simulink model "iff_sim"  (R2019b)
settings: Solver=VariableStepAuto  StartTime=0.0  StopTime=T  FixedStep=0.001  MaxStep=0.001  RelTol=1e-3
values from neighbouring files (symbols this model uses):
  bsc = 17    [model.mat]    (also in model_data.m)
  d_r = [0.01 0.01 0.01 0.01 0.01 0.01]    [model.mat]    (also in model_data.m = 0.01*ones(6,1))
  Fi_b_z = [0 2.09439510239 4.18879020479 1.0471975512 3.14159265359 5.23598775598]    [model.mat]    (also in model_data.m = [0;2/3;4/3;1/3;3/3;5/3]*pi)
  Fp = 148    [model.mat]    (also in model_data.m)
  ka = 11860000    [model.mat]    (also in model_data.m)
  Kd = 0    [ctc_data.m]
  Ki = 0    [ctc_data.m]
  Kp = 300    [ctc_data.m]
  ksc = 179000    [model.mat]    (also in model_data.m)
  l_r = [0.36 0.36 0.36 0.36 0.36 0.36]    [model.mat]    (also in model_data.m = 0.36*ones(6,1))
  la00 = 0.061    [model.mat]    (also in model_data.m)
  O_lb = [0 0 0 0 0 0]    [model.mat]    (also in model_data.m = [0;0;0;0;0;0])
  q_d = out_ik.q'    [ik_run.m]
  qt_d = out_ik.qt'    [ik_run.m]
  qtt_d = out_ik.qtt'    [ik_run.m]
  RMSforce = 35    [model.mat]
  s = out_ctc.s    [ctc_run.m]
  s_0 = s_d(:,:,1)    [ctc_run.m]    (also in iff_run.m)
  T = 1.5    [ctc_data.m]
  t_d = out_ik.t'    [ik_run.m]
  t_dist = 0.1    [model.mat]
  ts_noise = 1.6e-05    [model.mat]    (also in model_data.m)
  v_0 = v_d(:,:,1)    [ctc_run.m]    (also in iff_run.m)
  w_lb = 0.195    [model.mat]    (also in model_data.m)
  W_lb = 0.205    [model.mat]    (also in model_data.m)
  w_ub = 0.195    [model.mat]    (also in model_data.m)
  W_ub = 0.205    [model.mat]    (also in model_data.m)
undefined symbols (not defined in the file or in its folder): X, Y, Z
libraries: nesl_utility x282, sm_lib x208, dspindex x30, simulink x12, powerlib_meascontrol x1
(part 14 of 14)

== system iff_sim/High-authority control/CTC/computed torque control/bases + rods/upper base/O_ub -> H_4 ==
  rot z : sm_lib/Frames and Transforms/Rigid Transform  TranslationMethod=None  TranslationStandardOffset=0  TranslationLengthUnit=m  TranslationStandardAxis=+Z  TranslationCartesianOffset=[0 0 0]  TranslationROffset=0  TranslationROffsetUnits=m  TranslationZOffset=0  TranslationZOffsetUnits=m  TranslationThetaOffset=0  TranslationThetaOffsetUnits=deg  RotationMethod=StandardAxis  RotationAngleUnits=rad  RotationStandardAxis=+Z  RotationAngle=Fi_b_z(4)  RotationArbitraryAxis=[0 0 1]  FollAlignAxisA=+X  BaseAlignAxisA=+Y  FollAlignAxisB=+Y  BaseAlignAxisB=+Z  RotationSequenceAxes=FollowerAxes  RotationSequence=XYX  RotationSequenceAngles=[0 0 0]  RotationSequenceAnglesUnits=deg  RotationMatrix=[1 0 0; 0 1 0; 0 0 1]
  trans z : sm_lib/Frames and Transforms/Rigid Transform  TranslationMethod=StandardAxis  TranslationStandardOffset=h_ub  TranslationLengthUnit=m  TranslationStandardAxis=-Z  TranslationCartesianOffset=[0 0 0]  TranslationROffset=0  TranslationROffsetUnits=m  TranslationZOffset=0  TranslationZOffsetUnits=m  TranslationThetaOffset=0  TranslationThetaOffsetUnits=deg  RotationMethod=None  RotationAngleUnits=deg  RotationStandardAxis=+Z  RotationAngle=0.0  RotationArbitraryAxis=[0 0 1]  FollAlignAxisA=+X  BaseAlignAxisA=+Y  FollAlignAxisB=+Y  BaseAlignAxisB=+Z  RotationSequenceAxes=FollowerAxes  RotationSequence=XYX  RotationSequenceAngles=[0 0 0]  RotationSequenceAnglesUnits=deg  RotationMatrix=[1 0 0; 0 1 0; 0 0 1]
  transl y : sm_lib/Frames and Transforms/Rigid Transform  TranslationMethod=StandardAxis  TranslationStandardOffset=w_ub/2  TranslationLengthUnit=m  TranslationStandardAxis=+Y  TranslationCartesianOffset=[0 0 0]  TranslationROffset=0  TranslationROffsetUnits=m  TranslationZOffset=0  TranslationZOffsetUnits=m  TranslationThetaOffset=0  TranslationThetaOffsetUnits=deg  RotationMethod=None  RotationAngleUnits=deg  RotationStandardAxis=+Z  RotationAngle=0.0  RotationArbitraryAxis=[0 0 1]  FollAlignAxisA=+X  BaseAlignAxisA=+Y  FollAlignAxisB=+Y  BaseAlignAxisB=+Z  RotationSequenceAxes=FollowerAxes  RotationSequence=XYX  RotationSequenceAngles=[0 0 0]  RotationSequenceAnglesUnits=deg  RotationMatrix=[1 0 0; 0 1 0; 0 0 1]
  O_ub : PMIOPort  Side=Left
  H_4 : PMIOPort  Port=2  Side=Right
  connections:
  trans z/LConn1 -- O_ub/RConn1
  trans z/RConn1 -- rot z/LConn1
  transl y/LConn1 -- rot z/RConn1
  transl y/RConn1 -- H_4/RConn1

== system iff_sim/High-authority control/CTC/computed torque control/bases + rods/upper base/O_ub -> H_5 ==
  rot z : sm_lib/Frames and Transforms/Rigid Transform  TranslationMethod=None  TranslationStandardOffset=0  TranslationLengthUnit=m  TranslationStandardAxis=+Z  TranslationCartesianOffset=[0 0 0]  TranslationROffset=0  TranslationROffsetUnits=m  TranslationZOffset=0  TranslationZOffsetUnits=m  TranslationThetaOffset=0  TranslationThetaOffsetUnits=deg  RotationMethod=StandardAxis  RotationAngleUnits=rad  RotationStandardAxis=+Z  RotationAngle=Fi_b_z(5)  RotationArbitraryAxis=[0 0 1]  FollAlignAxisA=+X  BaseAlignAxisA=+Y  FollAlignAxisB=+Y  BaseAlignAxisB=+Z  RotationSequenceAxes=FollowerAxes  RotationSequence=XYX  RotationSequenceAngles=[0 0 0]  RotationSequenceAnglesUnits=deg  RotationMatrix=[1 0 0; 0 1 0; 0 0 1]
  trans z : sm_lib/Frames and Transforms/Rigid Transform  TranslationMethod=StandardAxis  TranslationStandardOffset=h_ub  TranslationLengthUnit=m  TranslationStandardAxis=-Z  TranslationCartesianOffset=[0 0 0]  TranslationROffset=0  TranslationROffsetUnits=m  TranslationZOffset=0  TranslationZOffsetUnits=m  TranslationThetaOffset=0  TranslationThetaOffsetUnits=deg  RotationMethod=None  RotationAngleUnits=deg  RotationStandardAxis=+Z  RotationAngle=0.0  RotationArbitraryAxis=[0 0 1]  FollAlignAxisA=+X  BaseAlignAxisA=+Y  FollAlignAxisB=+Y  BaseAlignAxisB=+Z  RotationSequenceAxes=FollowerAxes  RotationSequence=XYX  RotationSequenceAngles=[0 0 0]  RotationSequenceAnglesUnits=deg  RotationMatrix=[1 0 0; 0 1 0; 0 0 1]
  transl y : sm_lib/Frames and Transforms/Rigid Transform  TranslationMethod=StandardAxis  TranslationStandardOffset=w_ub/2  TranslationLengthUnit=m  TranslationStandardAxis=+Y  TranslationCartesianOffset=[0 0 0]  TranslationROffset=0  TranslationROffsetUnits=m  TranslationZOffset=0  TranslationZOffsetUnits=m  TranslationThetaOffset=0  TranslationThetaOffsetUnits=deg  RotationMethod=None  RotationAngleUnits=deg  RotationStandardAxis=+Z  RotationAngle=0.0  RotationArbitraryAxis=[0 0 1]  FollAlignAxisA=+X  BaseAlignAxisA=+Y  FollAlignAxisB=+Y  BaseAlignAxisB=+Z  RotationSequenceAxes=FollowerAxes  RotationSequence=XYX  RotationSequenceAngles=[0 0 0]  RotationSequenceAnglesUnits=deg  RotationMatrix=[1 0 0; 0 1 0; 0 0 1]
  O_ub : PMIOPort  Side=Left
  H_5 : PMIOPort  Port=2  Side=Right
  connections:
  trans z/LConn1 -- O_ub/RConn1
  trans z/RConn1 -- rot z/LConn1
  transl y/LConn1 -- rot z/RConn1
  transl y/RConn1 -- H_5/RConn1

== system iff_sim/High-authority control/CTC/computed torque control/bases + rods/upper base/O_ub -> H_6 ==
  rot z : sm_lib/Frames and Transforms/Rigid Transform  TranslationMethod=None  TranslationStandardOffset=0  TranslationLengthUnit=m  TranslationStandardAxis=+Z  TranslationCartesianOffset=[0 0 0]  TranslationROffset=0  TranslationROffsetUnits=m  TranslationZOffset=0  TranslationZOffsetUnits=m  TranslationThetaOffset=0  TranslationThetaOffsetUnits=deg  RotationMethod=StandardAxis  RotationAngleUnits=rad  RotationStandardAxis=+Z  RotationAngle=Fi_b_z(6)  RotationArbitraryAxis=[0 0 1]  FollAlignAxisA=+X  BaseAlignAxisA=+Y  FollAlignAxisB=+Y  BaseAlignAxisB=+Z  RotationSequenceAxes=FollowerAxes  RotationSequence=XYX  RotationSequenceAngles=[0 0 0]  RotationSequenceAnglesUnits=deg  RotationMatrix=[1 0 0; 0 1 0; 0 0 1]
  trans z : sm_lib/Frames and Transforms/Rigid Transform  TranslationMethod=StandardAxis  TranslationStandardOffset=h_ub  TranslationLengthUnit=m  TranslationStandardAxis=-Z  TranslationCartesianOffset=[0 0 0]  TranslationROffset=0  TranslationROffsetUnits=m  TranslationZOffset=0  TranslationZOffsetUnits=m  TranslationThetaOffset=0  TranslationThetaOffsetUnits=deg  RotationMethod=None  RotationAngleUnits=deg  RotationStandardAxis=+Z  RotationAngle=0.0  RotationArbitraryAxis=[0 0 1]  FollAlignAxisA=+X  BaseAlignAxisA=+Y  FollAlignAxisB=+Y  BaseAlignAxisB=+Z  RotationSequenceAxes=FollowerAxes  RotationSequence=XYX  RotationSequenceAngles=[0 0 0]  RotationSequenceAnglesUnits=deg  RotationMatrix=[1 0 0; 0 1 0; 0 0 1]
  transl y : sm_lib/Frames and Transforms/Rigid Transform  TranslationMethod=StandardAxis  TranslationStandardOffset=w_ub/2  TranslationLengthUnit=m  TranslationStandardAxis=+Y  TranslationCartesianOffset=[0 0 0]  TranslationROffset=0  TranslationROffsetUnits=m  TranslationZOffset=0  TranslationZOffsetUnits=m  TranslationThetaOffset=0  TranslationThetaOffsetUnits=deg  RotationMethod=None  RotationAngleUnits=deg  RotationStandardAxis=+Z  RotationAngle=0.0  RotationArbitraryAxis=[0 0 1]  FollAlignAxisA=+X  BaseAlignAxisA=+Y  FollAlignAxisB=+Y  BaseAlignAxisB=+Z  RotationSequenceAxes=FollowerAxes  RotationSequence=XYX  RotationSequenceAngles=[0 0 0]  RotationSequenceAnglesUnits=deg  RotationMatrix=[1 0 0; 0 1 0; 0 0 1]
  O_ub : PMIOPort  Side=Left
  H_6 : PMIOPort  Port=2  Side=Right
  connections:
  trans z/LConn1 -- O_ub/RConn1
  trans z/RConn1 -- rot z/LConn1
  transl y/LConn1 -- rot z/RConn1
  transl y/RConn1 -- H_6/RConn1

== matlab function iff_sim/High-authority control/CTC/computed torque control/bases + rods/v_r,v_ub -> v ==
  data: v_1 input; v output; v_2 input; v_3 input; v_4 input; v_5 input; v_6 input; v_ub input
function v = fcn(v_1,v_2,v_3,v_4,v_5,v_6,v_ub)
    v = [v_1,v_2,v_3,v_4,v_5,v_6,v_ub];
end

== matlab function iff_sim/dynamic model/v -> qt ==
  data: v input; qt output
function qt = fcn(v)
    qt = zeros(18,1);
    for r = 1:1:6
        qt(((r-1)*2+1):((r-1)*2+2),1) = v(4:5,r);
    end
    qt(13:end) = v(:,7);
end

== matlab function iff_sim/High-authority control/CTC/computed torque control/desired cable vectors// lengths/cable 2/cable force and length ==
  data: pz input; F_c output; fz input; l_c output
function [F_c,l_c] = fcn(pz,fz)
    if pz < 0 
        F_c = fz;
    else
        F_c = -fz;
    end
    l_c = abs(pz);
end

== matlab function iff_sim/dynamic model/rods + bases/s_r,s_ub -> s ==
  data: s_1 input; s output; s_2 input; s_3 input; s_4 input; s_5 input; s_6 input; s_ub input
function s = fcn(s_1,s_2,s_3,s_4,s_5,s_6,s_ub)
    s = [s_1,s_2,s_3,s_4,s_5,s_6,s_ub];
end

== matlab function iff_sim/dynamic model/rods + bases/v_r,v_ub -> v ==
  data: v_1 input; v output; v_2 input; v_3 input; v_4 input; v_5 input; v_6 input; v_ub input
function v = fcn(v_1,v_2,v_3,v_4,v_5,v_6,v_ub)
    v = [v_1,v_2,v_3,v_4,v_5,v_6,v_ub];
end

== matlab function iff_sim/High-authority control/CTC/computed torque control/desired cable vectors// lengths/cable 1/cable force and length ==
  data: pz input; F_c output; fz input; l_c output
function [F_c,l_c] = fcn(pz,fz)
    if pz < 0 
        F_c = fz;
    else
        F_c = -fz;
    end
    l_c = abs(pz);
end

== matlab function iff_sim/High-authority control/CTC/computed torque control/desired cable vectors// lengths/cable 3/cable force and length ==
  data: pz input; F_c output; fz input; l_c output
function [F_c,l_c] = fcn(pz,fz)
    if pz < 0 
        F_c = fz;
    else
        F_c = -fz;
    end
    l_c = abs(pz);
end

== matlab function iff_sim/High-authority control/CTC/computed torque control/desired cable vectors// lengths/cable 4/cable force and length ==
  data: pz input; F_c output; fz input; l_c output
function [F_c,l_c] = fcn(pz,fz)
    if pz < 0 
        F_c = fz;
    else
        F_c = -fz;
    end
    l_c = abs(pz);
end

== matlab function iff_sim/High-authority control/CTC/computed torque control/desired cable vectors// lengths/cable 5/cable force and length ==
  data: pz input; F_c output; fz input; l_c output
function [F_c,l_c] = fcn(pz,fz)
    if pz < 0 
        F_c = fz;
    else
        F_c = -fz;
    end
    l_c = abs(pz);
end

== matlab function iff_sim/High-authority control/CTC/computed torque control/desired cable vectors// lengths/cable 6/cable force and length ==
  data: pz input; F_c output; fz input; l_c output
function [F_c,l_c] = fcn(pz,fz)
    if pz < 0 
        F_c = fz;
    else
        F_c = -fz;
    end
    l_c = abs(pz);
end

== matlab function iff_sim/High-authority control/CTC/computed torque control/desired cable vectors// lengths/cable 7/cable force and length ==
  data: pz input; F_c output; fz input; l_c output
function [F_c,l_c] = fcn(pz,fz)
    if pz < 0 
        F_c = fz;
    else
        F_c = -fz;
    end
    l_c = abs(pz);
end

== matlab function iff_sim/High-authority control/CTC/computed torque control/desired cable vectors// lengths/cable 8/cable force and length ==
  data: pz input; F_c output; fz input; l_c output
function [F_c,l_c] = fcn(pz,fz)
    if pz < 0 
        F_c = fz;
    else
        F_c = -fz;
    end
    l_c = abs(pz);
end

== matlab function iff_sim/High-authority control/CTC/computed torque control/desired cable vectors// lengths/cable 9/cable force and length ==
  data: pz input; F_c output; fz input; l_c output
function [F_c,l_c] = fcn(pz,fz)
    if pz < 0 
        F_c = fz;
    else
        F_c = -fz;
    end
    l_c = abs(pz);
end

== matlab function iff_sim/High-authority control/CTC/computed torque control/desired cable vectors// lengths/cable 10/cable force and length ==
  data: pz input; F_c output; fz input; l_c output
function [F_c,l_c] = fcn(pz,fz)
    if pz < 0 
        F_c = fz;
    else
        F_c = -fz;
    end
    l_c = abs(pz);
end

== matlab function iff_sim/High-authority control/CTC/computed torque control/desired cable vectors// lengths/cable 11/cable force and length ==
  data: pz input; F_c output; fz input; l_c output
function [F_c,l_c] = fcn(pz,fz)
    if pz < 0 
        F_c = fz;
    else
        F_c = -fz;
    end
    l_c = abs(pz);
end

== matlab function iff_sim/High-authority control/CTC/computed torque control/desired cable vectors// lengths/cable 12/cable force and length ==
  data: pz input; F_c output; fz input; l_c output
function [F_c,l_c] = fcn(pz,fz)
    if pz < 0 
        F_c = fz;
    else
        F_c = -fz;
    end
    l_c = abs(pz);
end

== matlab function iff_sim/High-authority control/CTC/computed torque control/desired cable vectors// lengths/cable 13/cable force and length ==
  data: pz input; F_c output; fz input; l_c output
function [F_c,l_c] = fcn(pz,fz)
    if pz < 0 
        F_c = fz;
    else
        F_c = -fz;
    end
    l_c = abs(pz);
end

== matlab function iff_sim/High-authority control/CTC/computed torque control/desired cable vectors// lengths/cable 14/cable force and length ==
  data: pz input; F_c output; fz input; l_c output
function [F_c,l_c] = fcn(pz,fz)
    if pz < 0 
        F_c = fz;
    else
        F_c = -fz;
    end
    l_c = abs(pz);
end

== matlab function iff_sim/High-authority control/CTC/computed torque control/desired cable vectors// lengths/cable 15/cable force and length ==
  data: pz input; F_c output; fz input; l_c output
function [F_c,l_c] = fcn(pz,fz)
    if pz < 0 
        F_c = fz;
    else
        F_c = -fz;
    end
    l_c = abs(pz);
end

== matlab function iff_sim/High-authority control/CTC/computed torque control/desired cable vectors// lengths/cable 16/cable force and length ==
  data: pz input; F_c output; fz input; l_c output
function [F_c,l_c] = fcn(pz,fz)
    if pz < 0 
        F_c = fz;
    else
        F_c = -fz;
    end
    l_c = abs(pz);
end

== matlab function iff_sim/High-authority control/CTC/computed torque control/bases + rods/s_r,s_ub -> s ==
  data: s_1 input; s output; s_2 input; s_3 input; s_4 input; s_5 input; s_6 input; s_ub input
function s = fcn(s_1,s_2,s_3,s_4,s_5,s_6,s_ub)
    s = [s_1,s_2,s_3,s_4,s_5,s_6,s_ub];
end

== matlab function iff_sim/High-authority control/CTC/computed torque control/desired cable vectors// lengths/cable 17/cable force and length ==
  data: pz input; F_c output; fz input; l_c output
function [F_c,l_c] = fcn(pz,fz)
    if pz < 0 
        F_c = fz;
    else
        F_c = -fz;
    end
    l_c = abs(pz);
end

== matlab function iff_sim/dynamic model/s -> q ==
  data: s input; q output
function q = fcn(s)
    q = zeros(18,1);
    for r = 1:1:6
        q(((r-1)*2+1):((r-1)*2+2),1) = s(4:5,r);
    end
    q(13:end) = s(:,7);
end

== matlab function iff_sim/High-authority control/CTC/computed torque control/desired cable vectors// lengths/cable 18/cable force and length ==
  data: pz input; F_c output; fz input; l_c output
function [F_c,l_c] = fcn(pz,fz)
    if pz < 0 
        F_c = fz;
    else
        F_c = -fz;
    end
    l_c = abs(pz);
end
